simulink model "model_cosine_gust"  (R2020b)
settings: configuration reference "Configuration" (kept outside this file)
settings Model: Creator=dogukan  LastModifiedBy=dogukan
settings ConfigSetRef: SourceName=Configuration  SourceLocation=Base Workspace

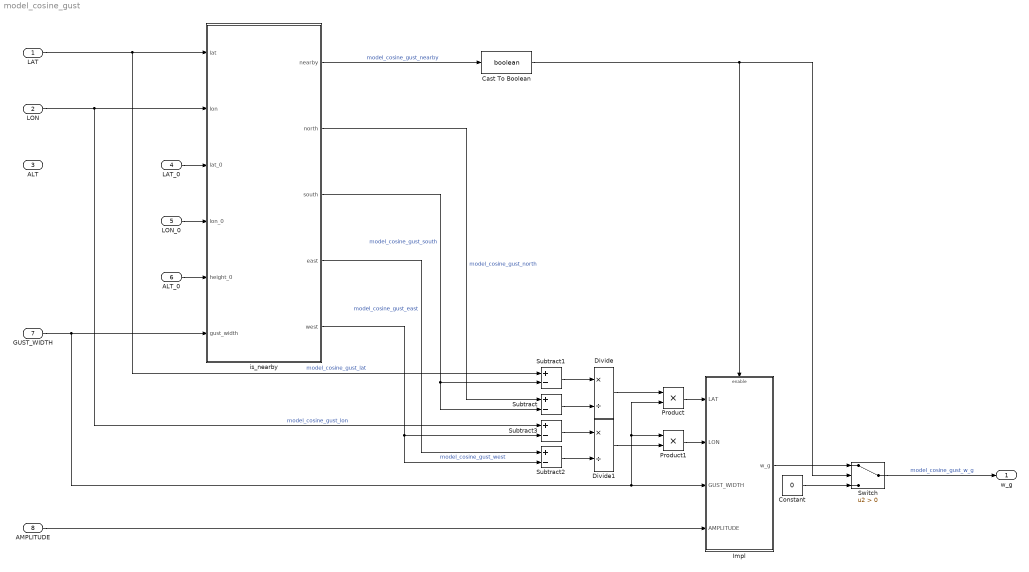
== system model_cosine_gust ==
  LAT : Inport
  LON : Inport  Port=2
  ALT : Inport  Port=3
  LAT_0 : Inport  Port=4
  LON_0 : Inport  Port=5
  ALT_0 : Inport  Port=6
  GUST_WIDTH : Inport  Port=7
  AMPLITUDE : Inport  Port=8
  Cast To Boolean : DataTypeConversion  OutDataTypeStr=boolean
  Constant : Constant  Value=0
  Divide : Product  Inputs=*/
  Divide1 : Product  Inputs=*/
  Impl : Subsystem  TreatAsAtomicUnit=on
  Product : Product
  Product1 : Product
  Subtract{,1..3} (4 alike) : Sum  Inputs=+-
  Switch : Switch  Criteria=u2 > Threshold
  is_nearby : MATLAB Function  TreatAsAtomicUnit=on
  w_g : Outport
  wires:
  LAT/1 -> is_nearby/1(lat), Subtract1/1  "model_cosine_gust_lat"
  LON/1 -> is_nearby/2(lon), Subtract3/1  "model_cosine_gust_lon"
  LAT_0/1 -> is_nearby/3(lat_0)
  LON_0/1 -> is_nearby/4(lon_0)
  ALT_0/1 -> is_nearby/5(height_0)
  is_nearby/1(nearby) -> Cast To Boolean/1  "model_cosine_gust_nearby"
  Constant/1 -> Switch/3
  Cast To Boolean/1 -> Switch/2, Impl/Enable
  Impl/1(w_g) -> Switch/1
  GUST_WIDTH/1 -> is_nearby/6(gust_width), Impl/3(GUST_WIDTH), Product1/1, Product/2
  AMPLITUDE/1 -> Impl/4(AMPLITUDE)
  Switch/1 -> w_g/1  "model_cosine_gust_w_g"
  is_nearby/2(north) -> Subtract/1  "model_cosine_gust_north"
  is_nearby/3(south) -> Subtract/2, Subtract1/2  "model_cosine_gust_south"
  Subtract1/1 -> Divide/1
  Subtract/1 -> Divide/2
  Divide/1 -> Product/1
  Product/1 -> Impl/1(LAT)
  is_nearby/4(east) -> Subtract2/1  "model_cosine_gust_east"
  is_nearby/5(west) -> Subtract2/2, Subtract3/2  "model_cosine_gust_west"
  Subtract3/1 -> Divide1/1
  Subtract2/1 -> Divide1/2
  Product1/1 -> Impl/2(LON)
  Divide1/1 -> Product1/2

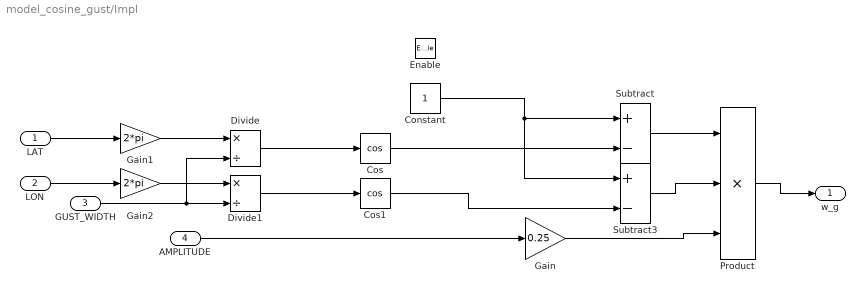
== system model_cosine_gust/Impl ==
  LAT : Inport
  LON : Inport  Port=2
  GUST_WIDTH : Inport  Port=3
  AMPLITUDE : Inport  Port=4
  Enable : EnablePort
  Constant : Constant
  Cos : Trigonometry  Operator=cos
  Cos1 : Trigonometry  Operator=cos
  Divide : Product  Inputs=*/
  Divide1 : Product  Inputs=*/
  Gain : Gain  Gain=0.25
  Gain1 : Gain  Gain=2*pi
  Gain2 : Gain  Gain=2*pi
  Product : Product  Inputs=3
  Subtract : Sum  Inputs=+-
  Subtract3 : Sum  Inputs=+-
  w_g : Outport
  wires:
  Product/1 -> w_g/1
  AMPLITUDE/1 -> Gain/1
  Gain/1 -> Product/3
  Constant/1 -> Subtract3/1, Subtract/1
  Cos/1 -> Subtract/2
  Cos1/1 -> Subtract3/2
  LAT/1 -> Gain1/1
  Gain1/1 -> Divide/1
  GUST_WIDTH/1 -> Divide/2, Divide1/2
  LON/1 -> Gain2/1
  Gain2/1 -> Divide1/1
  Divide/1 -> Cos/1
  Divide1/1 -> Cos1/1
  Subtract3/1 -> Product/2
  Subtract/1 -> Product/1

== matlab function model_cosine_gust/is_nearby ==
  data: lat input; nearby output; lon input; lat_0 input; lon_0 input; height_0 input; gust_width input; north output; south output; east output; west output
% model_sinusoidal_gust
function [nearby, north, south, east, west] = is_nearby(lat, lon, lat_0, lon_0, height_0, gust_width)
    % Units:
    % [lat] = rad
    % [lon] = rad
    % [lat_0] = rad
    % [lon_0] = rad
    % [height_0] = m
    % [gust_width] = m
    % Independet of altitude, phenomena is available on all heights, because otherwise height distribution is needed

    % Option 1: doesn't support code gen
    % [arclen, az] = distance(lat, lon, lat0, lon0);
    % nearby = arclen < width;

    % Option 2: ¯\_(ツ)_/¯
    % earth_radius = 6371000; % m
    % delta_phi = lat - lat_0;
    % delta_lambda = lon - lon_0;
    % a = sin(delta_phi / 2) ^ 2 + cos(lat) * cos(lat_0) * cos(delta_lambda / 2) ^ 2;
    % c = 2 * atan2(sqrt(a), sqrt(1 - a));
    % dist = earth_radius * c;
    % nearby = dist < width;

    % Option 3:
    north_lla = ned2lla([gust_width/2, 0, 0], [lat_0, lon_0, height_0], "flat");
    north = deg2rad(north_lla(1)); % rad
    south_lla = ned2lla([-gust_width/2, 0, 0], [lat_0, lon_0, height_0], "flat");
    south = deg2rad(south_lla(1)); % rad
    inside_lat = (south < lat) & (lat < north);
    % disp(inside_lat);

    east_lla = ned2lla([0, gust_width/2, 0], [lat_0, lon_0, height_0], "flat");
    east = deg2rad(east_lla(2)); % rad
    west_lla = ned2lla([0, -gust_width/2, 0], [lat_0, lon_0, height_0], "flat");
    west = deg2rad(west_lla(2)); % rad
    inside_lon = (west < lon) & (lon < east);
    % disp(inside_lon);

    nearby = inside_lat & inside_lon;
end
